simulink model "InertialSimulinkVariant"  (R2017a)
settings: Solver=VariableStepAuto  StartTime=0.0  StopTime=18  RelTol=1e-3
PreLoadFcn:
  | INERTIAL_REF_STEP=Simulink.Variant('REF_MODE==inertial_REF_TYPE.STEP')
  | INERTIAL_REF_SINE=Simulink.Variant('REF_MODE==inertial_REF_TYPE.SINE')
  | INERTIAL_REF_PULSE=Simulink.Variant('REF_MODE==inertial_REF_TYPE.PULSE')
  | 
  | INERTIAL_CTRL_EMPTY=Simulink.Variant('CTRL_MODE==inertial_CTRL_TYPE.EMPTY')
  | INERTIAL_CTRL_LINEAR=Simulink.Variant('CTRL_MODE==inertial_CTRL_TYPE.LINEAR')
  | INERTIAL_CTRL_NONLINEAR=Simulink.Variant('CTRL_MODE==inertial_CTRL_TYPE.NONLINEAR')
  | 
  | CTRL_MODE=inertial_CTRL_TYPE.EMPTY
  | REF_MODE=inertial_REF_TYPE.STEP
values from neighbouring files (symbols this model uses):
  c1 = 11    [InertialMatlab.m]
  c2 = 5    [InertialMatlab.m]
  d1 = 0.2    [InertialMatlab.m]
  d2 = 1.0    (= 1)    [InertialMatlab.m]
  J1 = 0.4    [InertialMatlab.m]
  J2 = 1.0    (= 1)    [InertialMatlab.m]
settings Model: Creator=mortenmj  LastModifiedBy=mortenmj

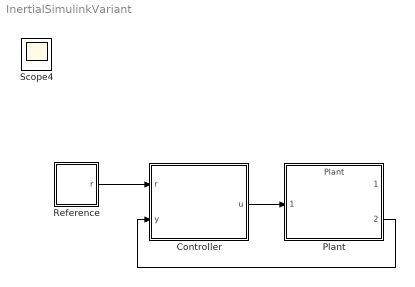
== system InertialSimulinkVariant ==
  Controller : Subsystem  Variant=on
      mask Display:
      | port_label('input', 1, 'r', 'interpreter', 'tex')
      | port_label('input', 2, '\omega', 'interpreter', 'tex')
      | port_label('output', 1, '\tau', 'interpreter', 'tex')
  Plant : ModelReference  ModelNameDialog=Plant  ParameterArgumentNames=J1,J2,c1,c2,d1,d2  ParameterArgumentValues=J1,J2,c1,c2,d1,d2  UsingDefaultArgumentValue=0,0,0,0,0,0  SimulationMode=Normal  ModelReferenceVersion=1.29  J1=J1  c1=c1  J2=J2  c2=c2  d1=d1  d2=d2
  Reference : Subsystem  Variant=on
      mask Display:
      | port_label('output', 1, 'r', 'interpreter', 'tex')
      | plot([0 1.5 3.5 5], [0 0 4 4])
  Scope4 : Scope
  wires:
  Reference/1(r) -> Controller/1(r)
  Controller/1(u) -> Plant/1
  Plant/2 -> Controller/2(y)

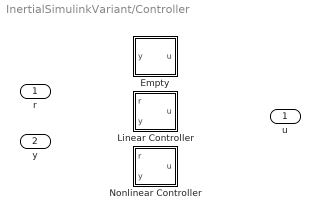
== system InertialSimulinkVariant/Controller ==
  r : Inport
  y : Inport  Port=2
  Empty : Subsystem  VariantControl=INERTIAL_CTRL_EMPTY
  Linear Controller : Subsystem  VariantControl=INERTIAL_CTRL_LINEAR
  Nonlinear Controller : Subsystem  VariantControl=INERTIAL_CTRL_NONLINEAR
  u : Outport

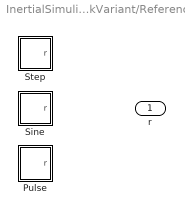
== system InertialSimulinkVariant/Reference ==
  Pulse : Subsystem  VariantControl=INERTIAL_REF_PULSE
  Sine : Subsystem  VariantControl=INERTIAL_REF_SINE
  Step : Subsystem  VariantControl=INERTIAL_REF_STEP
  r : Outport

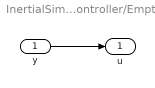
== system InertialSimulinkVariant/Controller/Empty ==
  y : Inport
  u : Outport
  wires:
  y/1 -> u/1

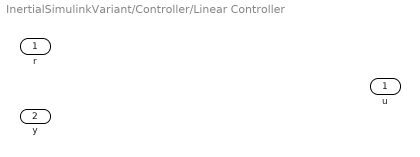
== system InertialSimulinkVariant/Controller/Linear Controller ==
  r : Inport
  y : Inport  Port=2
  u : Outport

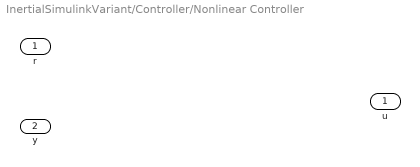
== system InertialSimulinkVariant/Controller/Nonlinear Controller ==
  r : Inport
  y : Inport  Port=2
  u : Outport

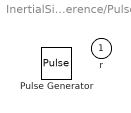
== system InertialSimulinkVariant/Reference/Pulse ==
  Pulse Generator : DiscretePulseGenerator  PulseType=Time based  Period=10  PulseWidth=5
  r : Outport

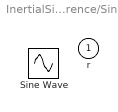
== system InertialSimulinkVariant/Reference/Sine ==
  Sine Wave : Sin  SampleTime=0
  r : Outport

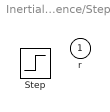
== system InertialSimulinkVariant/Reference/Step ==
  Step : Step  SampleTime=0
  r : Outport
